simulink model "rl_fwd"  (Simulink 7.5)
settings: Solver=ode45  StartTime=0.0  StopTime=0.5  RelTol=1e-3
undefined symbols (not defined in the file): deg
libraries: powerlib x13, powerlib_extras x4
settings Model: Creator=Singhal  LastModifiedBy=Singhal

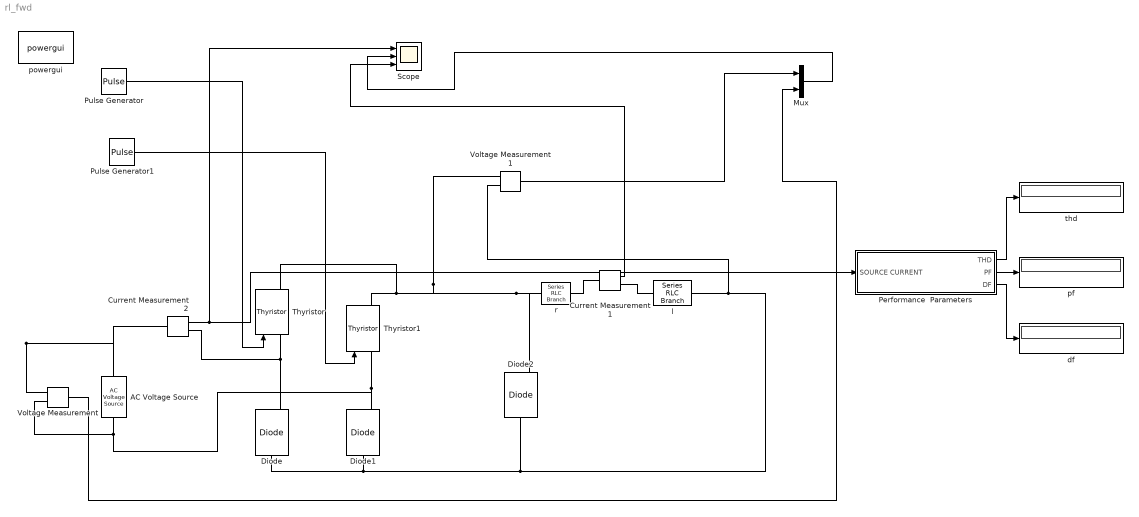
== system rl_fwd ==
  AC Voltage Source : powerlib/Electrical Sources/AC Voltage Source  DialogController=POWERSYS.PowerSysDialog  SystemSampleTime=-1  Amplitude=220  Phase=0  Frequency=50  SampleTime=0  Measurements=None
  Current Measurement1 : powerlib/Measurements/Current Measurement  DialogController=POWERSYS.PowerSysDialog  SystemSampleTime=-1  PhasorSimulation=off  OutputType=Complex  PSBequivalent=0
  Current Measurement2 : powerlib/Measurements/Current Measurement  DialogController=POWERSYS.PowerSysDialog  SystemSampleTime=-1  PhasorSimulation=off  OutputType=Complex  PSBequivalent=0
  Diode : powerlib/Power Electronics/Diode  DialogController=POWERSYS.PowerSysDialog  SystemSampleTime=-1  Ron=0.001  Lon=0  Vf=0.8  IC=0  UseSnubber=off  Rs=500  Cs=250e-9  Measurements=on
  Diode1 : powerlib/Power Electronics/Diode  DialogController=POWERSYS.PowerSysDialog  SystemSampleTime=-1  Ron=0.001  Lon=0  Vf=0.8  IC=0  UseSnubber=off  Rs=500  Cs=250e-9  Measurements=on
  Diode2 : powerlib/Power Electronics/Diode  DialogController=POWERSYS.PowerSysDialog  SystemSampleTime=-1  Ron=0.001  Lon=0  Vf=0.8  IC=0  UseSnubber=off  Rs=500  Cs=250e-9  Measurements=on
  Mux : Mux  Inputs=2
  Performance  Parameters : Subsystem
  Pulse Generator : DiscretePulseGenerator  PulseType=Time based  Amplitude=1  Period=0.02  PulseWidth=5  PhaseDelay=deg/18000  SampleTime=1
  Pulse Generator1 : DiscretePulseGenerator  PulseType=Time based  Amplitude=1  Period=0.02  PulseWidth=5  PhaseDelay=deg/18000+1/100  SampleTime=1
  Scope : Scope  NumInputPorts=3
      settings: YMin=-5~-5~-5  YMax=5~5~5
  Thyristor : powerlib/Power Electronics/Thyristor  DialogController=POWERSYS.PowerSysDialog  SystemSampleTime=-1  Ron=0.001  Lon=0  Vf=0.8  IC=0  Rs=500  Cs=250e-9  Measurements=on
  Thyristor1 : powerlib/Power Electronics/Thyristor  DialogController=POWERSYS.PowerSysDialog  SystemSampleTime=-1  Ron=0.001  Lon=0  Vf=0.8  IC=0  Rs=500  Cs=250e-9  Measurements=on
  Voltage Measurement : powerlib/Measurements/Voltage Measurement  DialogController=POWERSYS.PowerSysDialog  SystemSampleTime=-1  PhasorSimulation=off  OutputType=Complex  PSBequivalent=0
  Voltage Measurement1 : powerlib/Measurements/Voltage Measurement  DialogController=POWERSYS.PowerSysDialog  SystemSampleTime=-1  PhasorSimulation=off  OutputType=Complex  PSBequivalent=0
  df : Display
  l : powerlib/Elements/Series RLC Branch  DialogController=POWERSYS.PowerSysDialog  PhysicalDomain=powersysdomain  SubClassName=unknown  LeftPortType=p1  RightPortType=p1  LConnTagsString=__new0  RConnTagsString=__new0  BranchType=L  Resistance=1  Inductance=0.1  SetiL0=on  InitialCurrent=0  Capacitance=0  Setx0=off  InitialVoltage=0  Measurements=None
  pf : Display
  powergui : powerlib/powergui  Priority=1  SystemSampleTime=-1  SimulationMode=Discrete  SampleTime=50e-6  frequency=60  SPID=off  DisableSnubberDevices=off  DisableRonSwitches=off  DisableVfSwitches=off  SwTol=0  Interpol=off  frequencyindice=0  echomessages=off  HookPort=off  DisplayEquations=off  FunctionMessages=off  EnableUseOfTLC=off  x0status=blocks  RestoreLinks=warning  ResistiveCurrentMeasurement=off  Ylog=off  Xlog=on  ShowGrid=off  save=off  variable=ZData  ZoomFFT=off  StartTime=0.0  cycles=1  DisplayStyle=1  FreqAxis=off  MaxFrequency=1000  frequencyindicesteady=1  display=off  methode=off
  r : powerlib/Elements/Series RLC Branch  DialogController=POWERSYS.PowerSysDialog  PhysicalDomain=powersysdomain  SubClassName=unknown  LeftPortType=p1  RightPortType=p1  LConnTagsString=__new0  RConnTagsString=__new0  BranchType=R  Resistance=10  Inductance=1e-3  SetiL0=off  InitialCurrent=0  Capacitance=0  Setx0=off  InitialVoltage=0  Measurements=None
  thd : Display
  wires:
  Voltage Measurement/1 -> Mux/2
  Mux/1 -> Scope/2
  Pulse Generator1/1 -> Thyristor1/1
  Pulse Generator/1 -> Thyristor/1
  Current Measurement1/1 -> Scope/3
  Voltage Measurement1/1 -> Mux/1
  Current Measurement2/1 -> Performance  Parameters/1(SOURCE CURRENT), Scope/1
  Performance  Parameters/2(PF) -> pf/1
  Performance  Parameters/1(THD) -> thd/1
  Performance  Parameters/3(DF) -> df/1
  connections:
  Diode1/LConn1 -- Diode/LConn1 -- l/RConn1 -- Voltage Measurement1/LConn2 -- Diode2/LConn1
  r/LConn1 -- Voltage Measurement1/LConn1 -- Thyristor1/RConn1 -- Thyristor/RConn1 -- Diode2/RConn1
  Current Measurement2/RConn1 -- Diode/RConn1 -- Thyristor/LConn1
  Thyristor1/LConn1 -- Diode1/RConn1 -- AC Voltage Source/LConn1 -- Voltage Measurement/LConn2
  Current Measurement2/LConn1 -- Voltage Measurement/LConn1 -- AC Voltage Source/RConn1
  Current Measurement1/LConn1 -- r/RConn1
  Current Measurement1/RConn1 -- l/LConn1

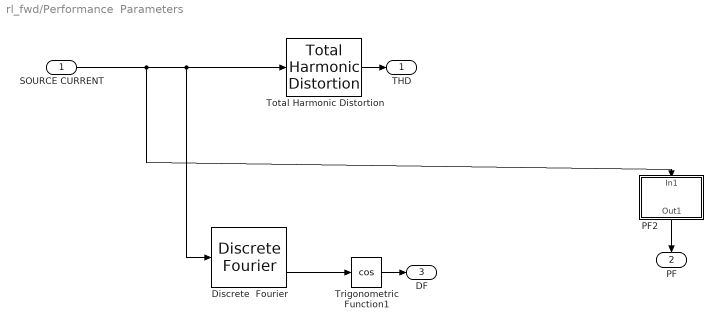
== system rl_fwd/Performance  Parameters ==
  SOURCE CURRENT : Inport
  Discrete  Fourier : powerlib_extras/Discrete Measurements/Discrete  Fourier  DialogController=POWERSYS.PowerSysDialog  SystemSampleTime=-1  Freq=50  n=1  Par_Init=[0 0]  Ts=50e-6
  PF2 : Subsystem
  Total Harmonic Distortion : powerlib_extras/Measurements/Total Harmonic Distortion  DialogController=POWERSYS.PowerSysDialog  SystemSampleTime=-1  f1=50
  Trigonometric Function1 : Trigonometry  Operator=cos
  THD : Outport
  PF : Outport  Port=2
  DF : Outport  Port=3
  wires:
  SOURCE CURRENT/1 -> PF2/1(In1), Discrete  Fourier/1, Total Harmonic Distortion/1
  Discrete  Fourier/2 -> Trigonometric Function1/1
  Total Harmonic Distortion/1 -> THD/1
  PF2/1(Out1) -> PF/1
  Trigonometric Function1/1 -> DF/1

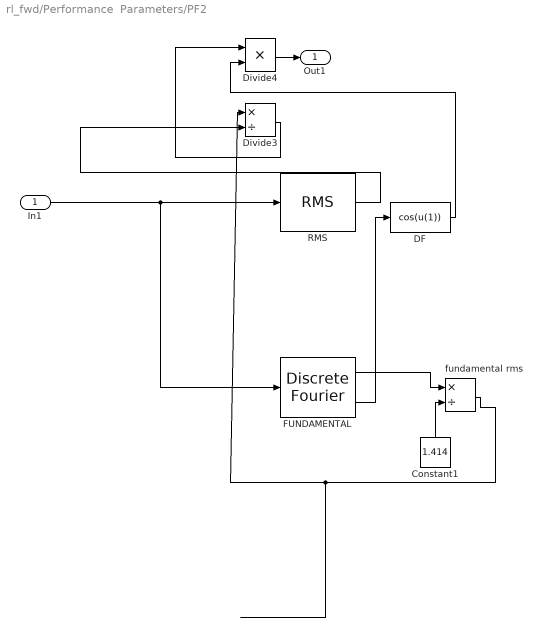
== system rl_fwd/Performance  Parameters/PF2 ==
  In1 : Inport
  Constant1 : Constant  Value=1.414  OutDataType=fixdt(1, 16)  OutScaling=2^0
  DF : Fcn  Expr=cos(u(1))
  Divide3 : Product  Inputs=*/  OutDataType=fixdt(1, 16)  OutScaling=2^-10
  Divide4 : Product  Inputs=**  OutDataType=fixdt(1, 16)  OutScaling=2^-10
  FUNDAMENTAL : powerlib_extras/Discrete Measurements/Discrete  Fourier  DialogController=POWERSYS.PowerSysDialog  SystemSampleTime=-1  Freq=50  n=1  Par_Init=[0 0]  Ts=50e-3
  RMS : powerlib_extras/Measurements/RMS  DialogController=POWERSYS.PowerSysDialog  SystemSampleTime=-1  f1=50
  fundamental rms : Product  Inputs=*/  OutDataType=fixdt(1, 16)  OutScaling=2^-10
  Out1 : Outport
  wires:
  DF/1 -> Divide4/2
  Divide3/1 -> Divide4/1
  fundamental rms/1 -> Divide3/1
  FUNDAMENTAL/1 -> fundamental rms/1
  FUNDAMENTAL/2 -> DF/1
  Constant1/1 -> fundamental rms/2
  Divide4/1 -> Out1/1
  In1/1 -> RMS/1, FUNDAMENTAL/1
  RMS/1 -> Divide3/2
